simulink model "Tra_TrqRed"  (R2016b)
settings: configuration reference "CodeGenConfigSet" (kept outside this file)
values from neighbouring files (symbols this model uses):
  Tra_trqDesMax_C = Calibration.Parameter    [init_Tra_TrqRed.m]
  Tra_trqDesMin_C = Calibration.Parameter    [init_Tra_TrqRed.m]
  Tra_trqLeadMax_C = Calibration.Parameter    [init_Tra_TrqRed.m]
  Tra_trqLeadMin_C = Calibration.Parameter    [init_Tra_TrqRed.m]
settings Model: Creator=Wollf  LastModifiedBy=lenovo
settings ConfigSetRef: SourceLocation=Base Workspace

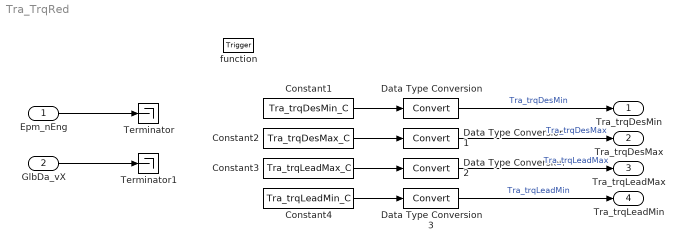
== system Tra_TrqRed ==
  Epm_nEng : Inport  Tag=rpm  Description=Engine speed  OutMin=0  OutMax=6000  OutDataTypeStr=EngSpeed_rpm
  GlbDa_vX : Inport  Tag=km/h  Description=Longitudinal vehicle speed (X-direction)  Port=2  OutMin=0  OutMax=250  OutDataTypeStr=VehSpeed_km_h
  function : TriggerPort  TriggerType=function-call  VariantControl=Variant
  Constant1 : Constant  Value=Tra_trqDesMin_C
  Constant2 : Constant  Value=Tra_trqDesMax_C
  Constant3 : Constant  Value=Tra_trqLeadMax_C
  Constant4 : Constant  Value=Tra_trqLeadMin_C
  Data Type Conversion{,1..3} (4 alike) : DataTypeConversion
  Terminator : Terminator
  Terminator1 : Terminator
  Tra_trqDesMin : Outport  Tag=Nm  Description=Increment torque demand from gearbox  OutMin=-3000  OutMax=3000  OutDataTypeStr=Trq_Nm
  Tra_trqDesMax : Outport  Tag=Nm  Description=Decrement torque demand from gearbox  Port=2  OutMin=-3000  OutMax=3000  OutDataTypeStr=Trq_Nm
  Tra_trqLeadMax : Outport  Tag=Nm  Description=decrement lead torque demand from gearbox  Port=3  OutMin=-3000  OutMax=3000  OutDataTypeStr=Trq_Nm
  Tra_trqLeadMin : Outport  Tag=Nm  Description=increment lead torque demand from gearbox  Port=4  OutMin=-3000  OutMax=3000  OutDataTypeStr=Trq_Nm
  wires:
  Constant1/1 -> Data Type Conversion/1
  Constant2/1 -> Data Type Conversion1/1
  Constant3/1 -> Data Type Conversion2/1
  Constant4/1 -> Data Type Conversion3/1
  Epm_nEng/1 -> Terminator/1
  GlbDa_vX/1 -> Terminator1/1
  Data Type Conversion/1 -> Tra_trqDesMin/1  "Tra_trqDesMin"
  Data Type Conversion1/1 -> Tra_trqDesMax/1  "Tra_trqDesMax"
  Data Type Conversion2/1 -> Tra_trqLeadMax/1  "Tra_trqLeadMax"
  Data Type Conversion3/1 -> Tra_trqLeadMin/1  "Tra_trqLeadMin"
